simulink model "ControladorPI2011"  (Simulink 7.7)
settings: Solver=ode45  SolverMode=SingleTasking  StartTime=0.0  StopTime=20.0  RelTol=1e-3
values from neighbouring files (symbols this model uses):
  C = [0.5 1 0]    [ExemploOgata.m]    (also in ProjetoControlPI.m = GYzss.C; dadosLab3.mat = [1 0]; ident.m = GYzss.C)
  F = FKi(1:size(G,2))    [ExemploOgata.m]    (also in ProjetoControlPI.m; dadosLab3.mat = [8860.59286484 122.620823611]; ident.m = acker(G, H, P))
  G = [0 1 0; 0 0 1; -0.12 -0.01 1]    [ExemploOgata.m]    (also in ProjetoControlPI.m = GYzss.A; dadosLab3.mat = [1  0.00945642354217; 0  0.893291168021]; ident.m = GYzss.A)
  H = [0;0;1]    [ExemploOgata.m]    (also in ProjetoControlPI.m = GYzss.B; dadosLab3.mat = [5.749068608e-05 0.0112859265204]; ident.m = GYzss.B)
  Kc = 1/Y(end)    [ExemploOgata.m]    (also in ProjetoControlPI.m; dadosLab3.mat = 0.000112859265204; ident.m = dcgain(SysCtl))
  Ki = FKi(size(G,2)+1:end)    [ExemploOgata.m]    (also in ProjetoControlPI.m)
  L = L'    [ProjetoControlPI.m]    (also in dadosLab3.mat = [1.89329116802 84.3838167047]; ident.m)
libraries: simulink x3
settings Model: Creator=castr  LastModifiedBy=castr  CovMetricSettings=dwe  CovHtmlReporting=off  covSaveCumulativeToWorkspaceVar=off  CovSaveSingleToWorkspaceVar=off  CovExternalEMLEnable=on
settings DataIOCC: LimitDataPoints=off  SaveFormat=StructureWithTime  SignalLoggingSaveFormat=Dataset
settings OptimizationCC: ExpressionDepthLimit=128
settings DebuggingCC: UnderspecifiedInitializationDetection=Simplified  MergeDetectMultiDrivingBlocksExec=error  SolverPrmCheckMsg=none  FcnCallInpInsideContextMsg=Enable All  StateNameClashWarn=none  SFUnexpectedBacktrackingDiag=error  SFNoUnconditionalDefaultTransitionDiag=error
settings HardwareCC: ProdBitPerPointer=64  ProdLargestAtomicFloat=Float  ProdIntDivRoundTo=Zero  ProdEndianess=LittleEndian  ProdHWDeviceType=Specified
settings CodeAppCC: CustomSymbolStrType=$N$R$M_T
settings GRTTargetCC: TargetFunctionLibrary=C99 (ISO)  GeneratePreprocessorConditionals=Use local settings

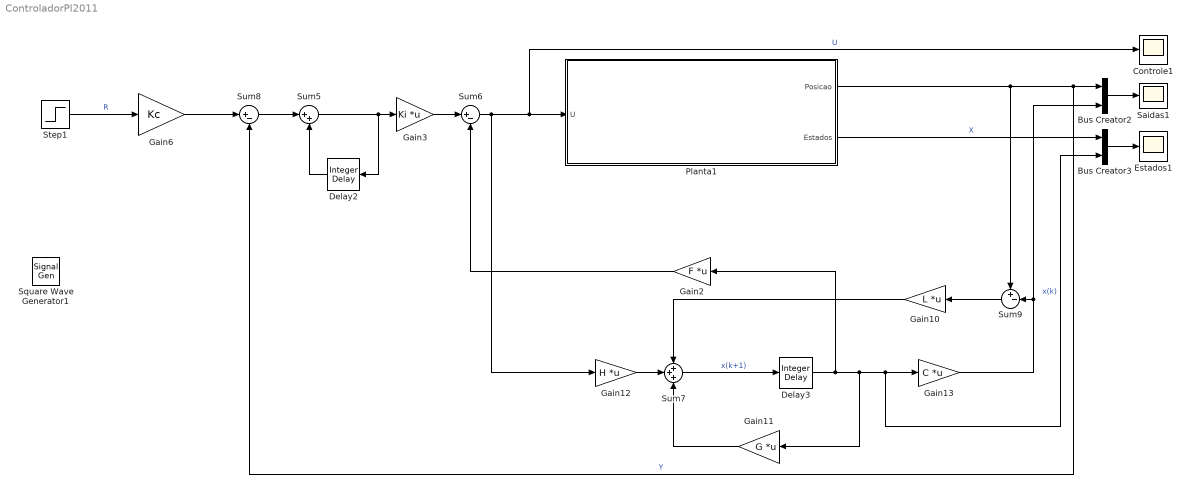
== system ControladorPI2011 ==
  Bus Creator2 : BusCreator  Inputs=2
  Bus Creator3 : BusCreator  Inputs=2
  Controle1 : Scope
      settings: TimeRange=auto  MaxDataPoints=5000  SaveToWorkspace=off  YMin=-1.18203  YMax=10.63706  SampleTime=-1
  Delay2 : simulink/Discrete/Integer Delay  NumDelays=1  vinit=0.0  samptime=-1
  Delay3 : simulink/Discrete/Integer Delay  NumDelays=1  vinit=0.0  samptime=Ts
  Estados1 : Scope
      settings: TimeRange=auto  MaxDataPoints=5000  SaveToWorkspace=off  SaveName=ScopeData2  YMin=-0.1692  YMax=1.5228  SampleTime=-1
  Gain10 : Gain  Gain=L  Multiplication=Matrix(K*u)
  Gain11 : Gain  Gain=G  Multiplication=Matrix(K*u)
  Gain12 : Gain  Gain=H  Multiplication=Matrix(K*u)
  Gain13 : Gain  Gain=C  Multiplication=Matrix(K*u)
  Gain2 : Gain  Gain=F  Multiplication=Matrix(K*u)
  Gain3 : Gain  Gain=Ki  Multiplication=Matrix(K*u)
  Gain6 : Gain  Gain=Kc
  Planta1 : Subsystem
  Saidas1 : Scope
      settings: TimeRange=auto  MaxDataPoints=5000  SaveToWorkspace=off  SaveName=ScopeData3  YMin=-2.7159  YMax=3.6351  SampleTime=-1
  Square Wave Generator1 : SignalGenerator  WaveForm=square  Units=rad/sec
  Step1 : Step  SampleTime=0
  Sum5 : Sum  Inputs=|++
  Sum6 : Sum  Inputs=|+-
  Sum7 : Sum  Inputs=+++
  Sum8 : Sum  Inputs=|+-
  Sum9 : Sum  Inputs=+-|
  wires:
  Step1/1 -> Gain6/1  "R"
  Gain6/1 -> Sum8/1
  Bus Creator2/1 -> Saidas1/1
  Gain11/1 -> Sum7/3
  Sum7/1 -> Delay3/1  "x(k+1)"
  Gain10/1 -> Sum7/1
  Gain3/1 -> Sum6/1
  Planta1/2(Estados) -> Bus Creator3/1  "X"
  Planta1/1(Posicao) -> Sum8/2, Bus Creator2/1, Sum9/1  "Y"
  Bus Creator3/1 -> Estados1/1
  Sum6/1 -> Gain12/1, Controle1/1, Planta1/1(U)  "U"
  Delay3/1 -> Gain2/1, Gain13/1, Bus Creator3/2, Gain11/1  "x(k)"
  Gain12/1 -> Sum7/2
  Delay2/1 -> Sum5/2
  Gain13/1 -> Sum9/2, Bus Creator2/2
  Sum9/1 -> Gain10/1
  Gain2/1 -> Sum6/2
  Sum8/1 -> Sum5/1
  Sum5/1 -> Delay2/1, Gain3/1

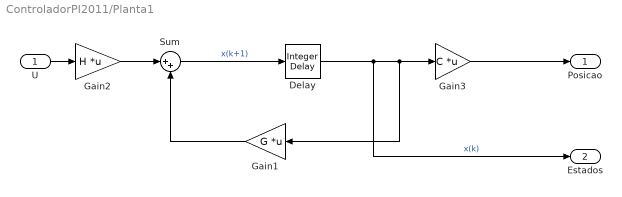
== system ControladorPI2011/Planta1 ==
  U : Inport
  Delay : simulink/Discrete/Integer Delay  NumDelays=1  vinit=[0 0]  samptime=Ts
  Gain1 : Gain  Gain=G  Multiplication=Matrix(K*u)
  Gain2 : Gain  Gain=H  Multiplication=Matrix(K*u)
  Gain3 : Gain  Gain=C  Multiplication=Matrix(K*u)
  Sum : Sum  Inputs=|++
  Posicao : Outport
  Estados : Outport  Port=2
  wires:
  Gain1/1 -> Sum/2
  Gain2/1 -> Sum/1
  U/1 -> Gain2/1
  Sum/1 -> Delay/1  "x(k+1)"
  Delay/1 -> Estados/1, Gain1/1, Gain3/1  "x(k)"
  Gain3/1 -> Posicao/1
